simulink library "IOBlock_Library_TTC580"  (R2021a)
settings: Solver=ode45  StartTime=0.0  StopTime=10.0  RelTol=1e-3
PreLoadFcn:
  | addpath(genpath(fileparts(which('IOBlock_Library_TTC580'))));
  | %addpath(genpath(fileparts(which('IOBlock_Library_TTC580.mdl'))))
  | try
  | addpath(genpath([fileparts(which('IOBlock_Library_TTC580')),'\..\DBC_Importer']));
  | addpath(genpath([fileparts(which('IOBlock_Library_TTC580')),'\..\EEPROM_Importer']));
  | addpath(genpath([fileparts(which('IOBlock_Library_TTC580')),'\..\UserDoc']));
  | catch
  | warning('IOBlock_Library_TTC580: add path to DBC_Importer and EEPROM_Importer manually');
  | end
  | try
  | if exist('..\CustomPackage\scripts\OpenAllPackages.m','file')
  |      run('..\CustomPackage\scripts\OpenAllPackages.m'); %always available, ggf. empty
  | end
  | catch
  | warning('A problem occurred opening automatically the CustomPackage. Please open libraries manually');
  | end
  | try
  | set_param(0,'EditorSmartEditingHotParam','off');
  | catch
  | warning('Simlink preferences for ''Edit key parameter when adding new blocks'' needs to be unchecked manually');
  | end
undefined symbols (not defined in the file or in its folder): ADC_Absolute_10V, ADC_Absolute_32V, ADC_Absolute_5V, ADC_BoardTemp, ADC_ChannelInit, ADC_Current, ADC_Get, ADC_K15_, ADC_Ratiometric_10V, ADC_Ratiometric_5V, ADC_Resistive, ADC_SensorSupply, ADC_UBAT, bit_packing, bit_unpacking, CAN_ConfigMsg, compare2error, compare2FET_PROT_REENABLE, crc32_calc_intern, CRC32_EEPROM_Read, CRC32_EEPROM_Write, DIAG_EnterSafestate, DIAG_Status, DIAG_Status_internal, EEPROM_Mirror, EEPROM_Read, EEPROM_Read_OffsetIn, EEPROM_Read_Raw, EEPROM_Write, EEPROM_Write_OffsetIn, EEPROM_Write_Raw, EnterSafestate, FPU_Handler, Get_DI, Get_DI_VarThreshold, Get_K15_, Get_Pulse_Freq_Curr, Get_Pulse_Freq_Volt, Get_WakeUp, GetDateAndTime, IO_ADC_ResetProtection, IO_Blk_Lib_TTC500, IO_CAN_ReadMsg, IO_CAN_WriteMsg, IO_DI_Get, IO_DI_Init, IO_DI_Init_Var, IO_DO_GetCur, IO_DO_GetVoltage, IO_DO_Init, IO_DO_ResetProtection, IO_DO_Set, IO_Driver_GetSerialNumber, IO_Driver_GetVersionOfDriver, IO_Driver_GetVersionOfFPGA, IO_EEPROM_GetStatus, IO_EEPROM_Init, IO_EEPROM_Read_raw, IO_EEPROM_Write, IO_EEPROM_Write_OffsetIn ... (+73)
libraries: simulink x43
(part 8 of 18)

== system IOBlock_Library_TTC580/ADC Blocks TTC580 IOlib/ADC_UBAT ==
  ADC_ChannelInit : Subsystem  LoadFcn=|  mask(ADC_ChannelInit_Code){SampleTime=-1, ttlib=IO_Blk_Lib_TTC500, ttDescription=ADC_ChannelInit, tt_iolib_version=0.19, adc_channel=adc_channel, adc_type=adc_type, range=range, pupd=pupd, sensor_supply=sensor_supply, safety_conf=NULL}
      | try
      | %
      | %Upgrade Information - standard BEGIN
      | new_color = 'blue';
      | new_ver = '0.19';
      | act_ver = get_param(gcb,'tt_iolib_version');
      | if not(strcmp(act_ver,new_ver))
      |     disp(['Upgrade block: ',gcb,char(10),'       Version: ',act_ver,' -> ',new_ver]);
      |     %switch - case for specific upgrade information e.g. additional parameter required 
      |     %Change appearance and version information
      |     set_param(gcb,'ForegroundColor',new_color);
      |     set_param(gcb,'tt_iolib_version',new_ver);
      | end
      | %Upgrade Information - standard END
      | catch
      | %Standard catch section BEGIN 
      | disp(' ');
      | disp('------------------------------------------------------------');
      | disp('An error occurred in a callback of the TTC580-BlockLib.');
      | disp(['Please check the parameters in the mask of ',gcb]);
      | disp('If you do not encounter any violations, then please '); 
      | disp('copy the following lines and report this to support@ttcontrol.com ');
      | disp('<< begin of error message dump >>');
      | disp(['Version of TTC580-BlockLib: ', get_param(gcb,'tt_iolib_version')]);
      | disp(get_param(gcb,'ttDescription'));
      | disp(gcb);
      | x=lasterror;disp(x.message);
      | disp(get_param(gcb,'MaskValues'));
      | disp(version);
      | disp(computer);
      | disp('<< end of error message dump >>');
      | disp('------------------------------------------------------------');
      | disp(' ');
      | %Standard catch section END
      | end
      mask help: Setup one ADC channel.
      mask init:
      | %
      settings: CopyFcn=%deleted
      mask Help: web(which('IO_ADC.h'))
      mask Callback adc_channel: %
      mask Callback adc_type: %
      mask Callback range: %
      mask Callback pupd: %
      mask Callback sensor_supply: %
      mask Callback safety_conf: %
  ADC_Get : Subsystem  LoadFcn=|  mask(ADC_Get_Code){SampleTime=-1, ttlib=IO_Blk_Lib_TTC500, ttDescription=ADC_Get, tt_iolib_version=0.19, adc_channel=adc_channel}
      | try
      | %
      | %Upgrade Information - standard BEGIN
      | new_color = 'blue';
      | new_ver = '0.19';
      | act_ver = get_param(gcb,'tt_iolib_version');
      | if not(strcmp(act_ver,new_ver))
      |     disp(['Upgrade block: ',gcb,char(10),'       Version: ',act_ver,' -> ',new_ver]);
      |     %switch - case for specific upgrade information e.g. additional parameter required 
      |     %Change appearance and version information
      |     set_param(gcb,'ForegroundColor',new_color);
      |     set_param(gcb,'tt_iolib_version',new_ver);
      | end
      | %Upgrade Information - standard END
      | catch
      | %Standard catch section BEGIN 
      | disp(' ');
      | disp('------------------------------------------------------------');
      | disp('An error occurred in a callback of the TTC580-BlockLib.');
      | disp(['Please check the parameters in the mask of ',gcb]);
      | disp('If you do not encounter any violations, then please '); 
      | disp('copy the following lines and report this to support@ttcontrol.com ');
      | disp('<< begin of error message dump >>');
      | disp(['Version of TTC580-BlockLib: ', get_param(gcb,'tt_iolib_version')]);
      | disp(get_param(gcb,'ttDescription'));
      | disp(gcb);
      | x=lasterror;disp(x.message);
      | disp(get_param(gcb,'MaskValues'));
      | disp(version);
      | disp(computer);
      | disp('<< end of error message dump >>');
      | disp('------------------------------------------------------------');
      | disp(' ');
      | %Standard catch section END
      | end
      mask help: Returns the value of the given ADC channel.
      mask init:
      | %
      settings: CopyFcn=%deleted
      mask Help: web(which('IO_ADC.h'))
      mask Callback adc_channel: %
  PWM_Init : Terminator
  PWM_Init1 : Terminator
  ErrorCode : Outport  VectorParamsAs1DForOutWhenUnconnected=off
  adc_value : Outport  Port=2  VectorParamsAs1DForOutWhenUnconnected=off
  wires:
  ADC_ChannelInit/1(ErrorCode) -> PWM_Init/1
  ADC_Get/3(fresh) -> PWM_Init1/1
  ADC_Get/1(ErrorCode) -> ErrorCode/1
  ADC_Get/2(adc_value) -> adc_value/1

== system IOBlock_Library_TTC580/CAN  Blocks TTC580 IOlib/ReadMsg_CAN ==
  note: Used as link in CAN-dbc Import Template
  note: IO_ErrorTypes may be exported
      | by adding Outports manually
  CAN_ConfigMsg : Subsystem  LoadFcn=|  mask(CAN_ConfigMsg_Code){SampleTime=-1, ttlib=IO_Blk_Lib_TTC500, ttDescription=CAN_ConfigMsg, tt_iolib_version=0.19, channel=channel, mode=mode, id_format=(id_format-1) %PopupNr - 1, id=id, ac_mask=['0x',dec2hex((id_format==1)*hex2dec('7FF')+(id_format==2)*hex2dec('1FFFFFFF')),'U']; %id_format = PopupNr}
      | try
      | %
      | %Upgrade Information - standard BEGIN
      | new_color = 'blue';
      | new_ver = '0.19';
      | act_ver = get_param(gcb,'tt_iolib_version');
      | if not(strcmp(act_ver,new_ver))
      |     disp(['Upgrade block: ',gcb,char(10),'       Version: ',act_ver,' -> ',new_ver]);
      |     %switch - case for specific upgrade information e.g. additional parameter required 
      |     %Change appearance and version information
      |     set_param(gcb,'ForegroundColor',new_color);
      |     set_param(gcb,'tt_iolib_version',new_ver);
      | end
      | %Upgrade Information - standard END
      | catch
      | %Standard catch section BEGIN 
      | disp(' ');
      | disp('------------------------------------------------------------');
      | disp('An error occurred in a callback of the TTC580-BlockLib.');
      | disp(['Please check the parameters in the mask of ',gcb]);
      | disp('If you do not encounter any violations, then please '); 
      | disp('copy the following lines and report this to support@ttcontrol.com ');
      | disp('<< begin of error message dump >>');
      | disp(['Version of TTC580-BlockLib: ', get_param(gcb,'tt_iolib_version')]);
      | disp(get_param(gcb,'ttDescription'));
      | disp(gcb);
      | x=lasterror;disp(x.message);
      | disp(get_param(gcb,'MaskValues'));
      | disp(version);
      | disp(computer);
      | disp('<< end of error message dump >>');
      | disp('------------------------------------------------------------');
      | disp(' ');
      | %Standard catch section END
      | end
      mask help: Configures a message object for the given CAN channel.
      mask init:
      | %
      settings: CopyFcn=%deleted
      mask Help: web(which('IO_CAN.h'))
      mask Callback channel: %
      mask Callback mode: %
      mask Callback id_format: %
      mask Callback id: %
      mask Callback ac_mask: %
  IO_CAN_ReadMsg : Subsystem  LoadFcn=|  mask(IO_CAN_ReadMsg_Code){SampleTime=-1, ttlib=IO_Blk_Lib_TTC500, ttDescription=IO_CAN_ReadMsg, tt_iolib_version=0.19}
      | try
      | %
      | %Upgrade Information - standard BEGIN
      | new_color = 'blue';
      | new_ver = '0.19';
      | act_ver = get_param(gcb,'tt_iolib_version');
      | if not(strcmp(act_ver,new_ver))
      |     disp(['Upgrade block: ',gcb,char(10),'       Version: ',act_ver,' -> ',new_ver]);
      |     %switch - case for specific upgrade information e.g. additional parameter required 
      |     %Change appearance and version information
      |     set_param(gcb,'ForegroundColor',new_color);
      |     set_param(gcb,'tt_iolib_version',new_ver);
      | end
      | %Upgrade Information - standard END
      | catch
      | %Standard catch section BEGIN 
      | disp(' ');
      | disp('------------------------------------------------------------');
      | disp('An error occurred in a callback of the TTC580-BlockLib.');
      | disp(['Please check the parameters in the mask of ',gcb]);
      | disp('If you do not encounter any violations, then please '); 
      | disp('copy the following lines and report this to support@ttcontrol.com ');
      | disp('<< begin of error message dump >>');
      | disp(['Version of TTC580-BlockLib: ', get_param(gcb,'tt_iolib_version')]);
      | disp(get_param(gcb,'ttDescription'));
      | disp(gcb);
      | x=lasterror;disp(x.message);
      | disp(get_param(gcb,'MaskValues'));
      | disp(version);
      | disp(computer);
      | disp('<< end of error message dump >>');
      | disp('------------------------------------------------------------');
      | disp(' ');
      | %Standard catch section END
      | end
      mask help: Reads a message from a given message object.
      mask init:
      | %
      settings: CopyFcn=%deleted
      mask Help: web(which('IO_CAN.h'))
  Terminator{2,6..8} (4 alike) : Terminator
  Read_Error : Outport  VectorParamsAs1DForOutWhenUnconnected=off
  data : Outport  Port=2  VectorParamsAs1DForOutWhenUnconnected=off
  wires:
  CAN_ConfigMsg/2(handle) -> IO_CAN_ReadMsg/1(handle)
  IO_CAN_ReadMsg/2(buffer_data) -> data/1
  IO_CAN_ReadMsg/5(buffer_id) -> Terminator6/1
  IO_CAN_ReadMsg/4(buffer_id_format) -> Terminator7/1
  IO_CAN_ReadMsg/3(buffer_length) -> Terminator8/1
  CAN_ConfigMsg/1(ErrorCode) -> Terminator2/1
  IO_CAN_ReadMsg/1(ErrorCode) -> Read_Error/1

== system IOBlock_Library_TTC580/CAN  Blocks TTC580 IOlib/ReadMsg_CAN_derated ==
  note: IO_ErrorTypes may be exported
      | by adding Outports manually
  CAN_ConfigMsg : Subsystem  LoadFcn=|  mask(CAN_ConfigMsg_Code){SampleTime=-1, ttlib=IO_Blk_Lib_TTC500, ttDescription=CAN_ConfigMsg, tt_iolib_version=0.19, channel=channel, mode=mode, id_format=(id_format-1) %PopupNr - 1, id=id, ac_mask=['0x',dec2hex((id_format==1)*hex2dec('7FF')+(id_format==2)*hex2dec('1FFFFFFF')),'U']; %id_format = PopupNr}
      | try
      | %
      | %Upgrade Information - standard BEGIN
      | new_color = 'blue';
      | new_ver = '0.19';
      | act_ver = get_param(gcb,'tt_iolib_version');
      | if not(strcmp(act_ver,new_ver))
      |     disp(['Upgrade block: ',gcb,char(10),'       Version: ',act_ver,' -> ',new_ver]);
      |     %switch - case for specific upgrade information e.g. additional parameter required 
      |     %Change appearance and version information
      |     set_param(gcb,'ForegroundColor',new_color);
      |     set_param(gcb,'tt_iolib_version',new_ver);
      | end
      | %Upgrade Information - standard END
      | catch
      | %Standard catch section BEGIN 
      | disp(' ');
      | disp('------------------------------------------------------------');
      | disp('An error occurred in a callback of the TTC580-BlockLib.');
      | disp(['Please check the parameters in the mask of ',gcb]);
      | disp('If you do not encounter any violations, then please '); 
      | disp('copy the following lines and report this to support@ttcontrol.com ');
      | disp('<< begin of error message dump >>');
      | disp(['Version of TTC580-BlockLib: ', get_param(gcb,'tt_iolib_version')]);
      | disp(get_param(gcb,'ttDescription'));
      | disp(gcb);
      | x=lasterror;disp(x.message);
      | disp(get_param(gcb,'MaskValues'));
      | disp(version);
      | disp(computer);
      | disp('<< end of error message dump >>');
      | disp('------------------------------------------------------------');
      | disp(' ');
      | %Standard catch section END
      | end
      mask help: Configures a message object for the given CAN channel.
      mask init:
      | %
      settings: CopyFcn=%deleted
      mask Help: web(which('IO_CAN.h'))
      mask Callback channel: %
      mask Callback mode: %
      mask Callback id_format: %
      mask Callback id: %
      mask Callback ac_mask: %
  IO_CAN_ReadMsg_x : Subsystem  LoadFcn=|  mask(IO_CAN_ReadMsg_Code){SampleTime=-1, ttlib=IO_Blk_Lib_TTC500, ttDescription=IO_CAN_ReadMsg, tt_iolib_version=0.19}
      | try
      | %
      | %Upgrade Information - standard BEGIN
      | new_color = 'blue';
      | new_ver = '0.19';
      | act_ver = get_param(gcb,'tt_iolib_version');
      | if not(strcmp(act_ver,new_ver))
      |     disp(['Upgrade block: ',gcb,char(10),'       Version: ',act_ver,' -> ',new_ver]);
      |     %switch - case for specific upgrade information e.g. additional parameter required 
      |     %Change appearance and version information
      |     set_param(gcb,'ForegroundColor',new_color);
      |     set_param(gcb,'tt_iolib_version',new_ver);
      | end
      | %Upgrade Information - standard END
      | catch
      | %Standard catch section BEGIN 
      | disp(' ');
      | disp('------------------------------------------------------------');
      | disp('An error occurred in a callback of the TTC580-BlockLib.');
      | disp(['Please check the parameters in the mask of ',gcb]);
      | disp('If you do not encounter any violations, then please '); 
      | disp('copy the following lines and report this to support@ttcontrol.com ');
      | disp('<< begin of error message dump >>');
      | disp(['Version of TTC580-BlockLib: ', get_param(gcb,'tt_iolib_version')]);
      | disp(get_param(gcb,'ttDescription'));
      | disp(gcb);
      | x=lasterror;disp(x.message);
      | disp(get_param(gcb,'MaskValues'));
      | disp(version);
      | disp(computer);
      | disp('<< end of error message dump >>');
      | disp('------------------------------------------------------------');
      | disp(' ');
      | %Standard catch section END
      | end
      mask help: Reads a message from a given message object.
      mask init:
      | %
      settings: CopyFcn=%deleted
      mask Help: web(which('IO_CAN.h'))
  Terminator{2,6..8} (4 alike) : Terminator
  Trigger : Subsystem  mask(Derate Trigger){derate=derate}
      mask help: derate "n": every n-th cylce a trigger is submitted
  Read_Error_debcd : Outport  VectorParamsAs1DForOutWhenUnconnected=off
  data : Outport  Port=2  VectorParamsAs1DForOutWhenUnconnected=off
  wires:
  IO_CAN_ReadMsg_x/1(ErrorCode) -> Read_Error_debcd/1
  CAN_ConfigMsg/1(ErrorCode) -> Terminator2/1
  IO_CAN_ReadMsg_x/3(buffer_length) -> Terminator8/1
  IO_CAN_ReadMsg_x/4(buffer_id_format) -> Terminator7/1
  IO_CAN_ReadMsg_x/5(buffer_id) -> Terminator6/1
  IO_CAN_ReadMsg_x/2(buffer_data) -> data/1
  CAN_ConfigMsg/2(handle) -> IO_CAN_ReadMsg_x/1(handle)
  Trigger/1(Trigger) -> IO_CAN_ReadMsg_x/Enable

== system IOBlock_Library_TTC580/CAN  Blocks TTC580 IOlib/WriteMsg_CAN ==
  note: IO_ErrorTypes may be exported
      | by adding Outports manually
  note: Used as link in CAN-dbc Import Template
  data : Inport
  CAN_ConfigMsg : Subsystem  LoadFcn=|  mask(CAN_ConfigMsg_Code){SampleTime=-1, ttlib=IO_Blk_Lib_TTC500, ttDescription=CAN_ConfigMsg, tt_iolib_version=0.19, channel=channel, mode=mode, id_format=(id_format-1) %PopupNr - 1, id=id, ac_mask=['0x',dec2hex((id_format==1)*hex2dec('7FF')+(id_format==2)*hex2dec('1FFFFFFF')),'U']; %id_format = PopupNr}
      | try
      | %
      | %Upgrade Information - standard BEGIN
      | new_color = 'blue';
      | new_ver = '0.19';
      | act_ver = get_param(gcb,'tt_iolib_version');
      | if not(strcmp(act_ver,new_ver))
      |     disp(['Upgrade block: ',gcb,char(10),'       Version: ',act_ver,' -> ',new_ver]);
      |     %switch - case for specific upgrade information e.g. additional parameter required 
      |     %Change appearance and version information
      |     set_param(gcb,'ForegroundColor',new_color);
      |     set_param(gcb,'tt_iolib_version',new_ver);
      | end
      | %Upgrade Information - standard END
      | catch
      | %Standard catch section BEGIN 
      | disp(' ');
      | disp('------------------------------------------------------------');
      | disp('An error occurred in a callback of the TTC580-BlockLib.');
      | disp(['Please check the parameters in the mask of ',gcb]);
      | disp('If you do not encounter any violations, then please '); 
      | disp('copy the following lines and report this to support@ttcontrol.com ');
      | disp('<< begin of error message dump >>');
      | disp(['Version of TTC580-BlockLib: ', get_param(gcb,'tt_iolib_version')]);
      | disp(get_param(gcb,'ttDescription'));
      | disp(gcb);
      | x=lasterror;disp(x.message);
      | disp(get_param(gcb,'MaskValues'));
      | disp(version);
      | disp(computer);
      | disp('<< end of error message dump >>');
      | disp('------------------------------------------------------------');
      | disp(' ');
      | %Standard catch section END
      | end
      mask help: Configures a message object for the given CAN channel.
      mask init:
      | %
      settings: CopyFcn=%deleted
      mask Help: web(which('IO_CAN.h'))
      mask Callback channel: %
      mask Callback mode: %
      mask Callback id_format: %
      mask Callback id: %
      mask Callback ac_mask: %
  IO_CAN_WriteMsg : Subsystem  LoadFcn=|  mask(IO_CAN_WriteMsg_Code){SampleTime=-1, ttlib=IO_Blk_Lib_TTC500, ttDescription=IO_CAN_WriteMsg, tt_iolib_version=0.19}
      | try
      | %
      | %Upgrade Information - standard BEGIN
      | new_color = 'blue';
      | new_ver = '0.19';
      | act_ver = get_param(gcb,'tt_iolib_version');
      | if not(strcmp(act_ver,new_ver))
      |     disp(['Upgrade block: ',gcb,char(10),'       Version: ',act_ver,' -> ',new_ver]);
      |     %switch - case for specific upgrade information e.g. additional parameter required 
      |     %Change appearance and version information
      |     set_param(gcb,'ForegroundColor',new_color);
      |     set_param(gcb,'tt_iolib_version',new_ver);
      | end
      | %Upgrade Information - standard END
      | catch
      | %Standard catch section BEGIN 
      | disp(' ');
      | disp('------------------------------------------------------------');
      | disp('An error occurred in a callback of the TTC580-BlockLib.');
      | disp(['Please check the parameters in the mask of ',gcb]);
      | disp('If you do not encounter any violations, then please '); 
      | disp('copy the following lines and report this to support@ttcontrol.com ');
      | disp('<< begin of error message dump >>');
      | disp(['Version of TTC580-BlockLib: ', get_param(gcb,'tt_iolib_version')]);
      | disp(get_param(gcb,'ttDescription'));
      | disp(gcb);
      | x=lasterror;disp(x.message);
      | disp(get_param(gcb,'MaskValues'));
      | disp(version);
      | disp(computer);
      | disp('<< end of error message dump >>');
      | disp('------------------------------------------------------------');
      | disp(' ');
      | %Standard catch section END
      | end
      mask help: Transmits a CAN message, using the given channel and message object.
      mask init:
      | %
      settings: CopyFcn=%deleted
      mask Help: web(which('IO_CAN.h'))
  Terminator2 : Terminator
  id_TX : Constant  Value=id  OutDataTypeStr=uint32
  id_format_TX : Constant  Value=(id_format - 1) %=PopupEntryNr - 1  OutDataTypeStr=Inherit: Inherit via back propagation
  length_TX : Constant  Value=length  OutDataTypeStr=Inherit: Inherit via back propagation
  Write_Error : Outport  VectorParamsAs1DForOutWhenUnconnected=off
  wires:
  CAN_ConfigMsg/1(ErrorCode) -> Terminator2/1
  IO_CAN_WriteMsg/1(ErrorCode) -> Write_Error/1
  CAN_ConfigMsg/2(handle) -> IO_CAN_WriteMsg/1(handle)
  data/1 -> IO_CAN_WriteMsg/2(buffer_data)
  length_TX/1 -> IO_CAN_WriteMsg/3(buffer_length)
  id_format_TX/1 -> IO_CAN_WriteMsg/4(buffer_id_format)
  id_TX/1 -> IO_CAN_WriteMsg/5(buffer_id)

== system IOBlock_Library_TTC580/CAN  Blocks TTC580 IOlib/WriteMsg_CAN_derated ==
  note: IO_ErrorTypes may be exported
      | by adding Outports manually
  data : Inport
  CAN_ConfigMsg : Subsystem  LoadFcn=|  mask(CAN_ConfigMsg_Code){SampleTime=-1, ttlib=IO_Blk_Lib_TTC500, ttDescription=CAN_ConfigMsg, tt_iolib_version=0.19, channel=channel, mode=mode, id_format=(id_format-1) %PopupNr - 1, id=id, ac_mask=['0x',dec2hex((id_format==1)*hex2dec('7FF')+(id_format==2)*hex2dec('1FFFFFFF')),'U']; %id_format = PopupNr}
      | try
      | %
      | %Upgrade Information - standard BEGIN
      | new_color = 'blue';
      | new_ver = '0.19';
      | act_ver = get_param(gcb,'tt_iolib_version');
      | if not(strcmp(act_ver,new_ver))
      |     disp(['Upgrade block: ',gcb,char(10),'       Version: ',act_ver,' -> ',new_ver]);
      |     %switch - case for specific upgrade information e.g. additional parameter required 
      |     %Change appearance and version information
      |     set_param(gcb,'ForegroundColor',new_color);
      |     set_param(gcb,'tt_iolib_version',new_ver);
      | end
      | %Upgrade Information - standard END
      | catch
      | %Standard catch section BEGIN 
      | disp(' ');
      | disp('------------------------------------------------------------');
      | disp('An error occurred in a callback of the TTC580-BlockLib.');
      | disp(['Please check the parameters in the mask of ',gcb]);
      | disp('If you do not encounter any violations, then please '); 
      | disp('copy the following lines and report this to support@ttcontrol.com ');
      | disp('<< begin of error message dump >>');
      | disp(['Version of TTC580-BlockLib: ', get_param(gcb,'tt_iolib_version')]);
      | disp(get_param(gcb,'ttDescription'));
      | disp(gcb);
      | x=lasterror;disp(x.message);
      | disp(get_param(gcb,'MaskValues'));
      | disp(version);
      | disp(computer);
      | disp('<< end of error message dump >>');
      | disp('------------------------------------------------------------');
      | disp(' ');
      | %Standard catch section END
      | end
      mask help: Configures a message object for the given CAN channel.
      mask init:
      | %
      settings: CopyFcn=%deleted
      mask Help: web(which('IO_CAN.h'))
      mask Callback channel: %
      mask Callback mode: %
      mask Callback id_format: %
      mask Callback id: %
      mask Callback ac_mask: %
  IO_CAN_WriteMsg_x : Subsystem  LoadFcn=|  mask(IO_CAN_WriteMsg_Code){SampleTime=-1, ttlib=IO_Blk_Lib_TTC500, ttDescription=IO_CAN_WriteMsg, tt_iolib_version=0.19}
      | try
      | %
      | %Upgrade Information - standard BEGIN
      | new_color = 'blue';
      | new_ver = '0.19';
      | act_ver = get_param(gcb,'tt_iolib_version');
      | if not(strcmp(act_ver,new_ver))
      |     disp(['Upgrade block: ',gcb,char(10),'       Version: ',act_ver,' -> ',new_ver]);
      |     %switch - case for specific upgrade information e.g. additional parameter required 
      |     %Change appearance and version information
      |     set_param(gcb,'ForegroundColor',new_color);
      |     set_param(gcb,'tt_iolib_version',new_ver);
      | end
      | %Upgrade Information - standard END
      | catch
      | %Standard catch section BEGIN 
      | disp(' ');
      | disp('------------------------------------------------------------');
      | disp('An error occurred in a callback of the TTC580-BlockLib.');
      | disp(['Please check the parameters in the mask of ',gcb]);
      | disp('If you do not encounter any violations, then please '); 
      | disp('copy the following lines and report this to support@ttcontrol.com ');
      | disp('<< begin of error message dump >>');
      | disp(['Version of TTC580-BlockLib: ', get_param(gcb,'tt_iolib_version')]);
      | disp(get_param(gcb,'ttDescription'));
      | disp(gcb);
      | x=lasterror;disp(x.message);
      | disp(get_param(gcb,'MaskValues'));
      | disp(version);
      | disp(computer);
      | disp('<< end of error message dump >>');
      | disp('------------------------------------------------------------');
      | disp(' ');
      | %Standard catch section END
      | end
      mask help: Transmits a CAN message, using the given channel and message object.
      mask init:
      | %
      settings: CopyFcn=%deleted
      mask Help: web(which('IO_CAN.h'))
  Terminator2 : Terminator
  Trigger : Subsystem  mask(Derate Trigger){derate=derate}
      mask help: derate "n": every n-th cylce a trigger is submitted
  id_TX : Constant  Value=id  OutDataTypeStr=uint32
  id_format_TX : Constant  Value=(id_format - 1) %=PopupEntryNr - 1  OutDataTypeStr=Inherit: Inherit via back propagation
  length_TX : Constant  Value=length  OutDataTypeStr=Inherit: Inherit via back propagation
  Write_Error : Outport  VectorParamsAs1DForOutWhenUnconnected=off
  wires:
  Trigger/1(Trigger) -> IO_CAN_WriteMsg_x/Enable
  id_TX/1 -> IO_CAN_WriteMsg_x/5(buffer_id)
  id_format_TX/1 -> IO_CAN_WriteMsg_x/4(buffer_id_format)
  length_TX/1 -> IO_CAN_WriteMsg_x/3(buffer_length)
  data/1 -> IO_CAN_WriteMsg_x/2(buffer_data)
  CAN_ConfigMsg/2(handle) -> IO_CAN_WriteMsg_x/1(handle)
  IO_CAN_WriteMsg_x/1(ErrorCode) -> Write_Error/1
  CAN_ConfigMsg/1(ErrorCode) -> Terminator2/1

== system IOBlock_Library_TTC580/CAN  Blocks TTC580 IOlib/bit_packing ==
  Data_in : Inport
  bit_packing_s : S-Function  FunctionName=bit_packing_s  Parameters=SampleTime,Endianness,Format,Inversion,Startbit,Width_bits,Factor,Offset  SFunctionDeploymentMode=off  EnableBusSupport=off
  Data_out : Outport  VectorParamsAs1DForOutWhenUnconnected=off
  wires:
  bit_packing_s/1 -> Data_out/1
  Data_in/1 -> bit_packing_s/1

== system IOBlock_Library_TTC580/CAN  Blocks TTC580 IOlib/bit_unpacking ==
  Data_in : Inport
  bit_unpacking_s : S-Function  FunctionName=bit_unpacking_s  Parameters=SampleTime,Endianness,Format,Inversion,Startbit,Width_bits,Factor,Offset  SFunctionDeploymentMode=off  EnableBusSupport=off
  Data_out : Outport  VectorParamsAs1DForOutWhenUnconnected=off
  wires:
  bit_unpacking_s/1 -> Data_out/1
  Data_in/1 -> bit_unpacking_s/1

== system IOBlock_Library_TTC580/DIO Blocks TTC580 IOlib/Get_DI ==
  IO_DI_Get : Subsystem  LoadFcn=|  mask(IO_DI_Get_Code){SampleTime=-1, ttlib=IO_Blk_Lib_TTC500, ttDescription=IO_DI_Get, tt_iolib_version=0.19, di_channel=di_channel}
      | try
      | %
      | %Upgrade Information - standard BEGIN
      | new_color = 'blue';
      | new_ver = '0.19';
      | act_ver = get_param(gcb,'tt_iolib_version');
      | if not(strcmp(act_ver,new_ver))
      |     disp(['Upgrade block: ',gcb,char(10),'       Version: ',act_ver,' -> ',new_ver]);
      |     %switch - case for specific upgrade information e.g. additional parameter required 
      |     %Change appearance and version information
      |     set_param(gcb,'ForegroundColor',new_color);
      |     set_param(gcb,'tt_iolib_version',new_ver);
      | end
      | %Upgrade Information - standard END
      | catch
      | %Standard catch section BEGIN 
      | disp(' ');
      | disp('------------------------------------------------------------');
      | disp('An error occurred in a callback of the TTC580-BlockLib.');
      | disp(['Please check the parameters in the mask of ',gcb]);
      | disp('If you do not encounter any violations, then please '); 
      | disp('copy the following lines and report this to support@ttcontrol.com ');
      | disp('<< begin of error message dump >>');
      | disp(['Version of TTC580-BlockLib: ', get_param(gcb,'tt_iolib_version')]);
      | disp(get_param(gcb,'ttDescription'));
      | disp(gcb);
      | x=lasterror;disp(x.message);
      | disp(get_param(gcb,'MaskValues'));
      | disp(version);
      | disp(computer);
      | disp('<< end of error message dump >>');
      | disp('------------------------------------------------------------');
      | disp(' ');
      | %Standard catch section END
      | end
      mask help: Gets the value of a digital input.
      mask init:
      | %
      settings: CopyFcn=%deleted
      mask Help: web(which('IO_DIO.h'))
      mask Callback di_channel: %
  IO_DI_Init : Subsystem  LoadFcn=|  mask(IO_DI_Init_Code){SampleTime=-1, ttlib=IO_Blk_Lib_TTC500, ttDescription=IO_DI_Init, tt_iolib_version=0.19, di_channel=di_channel, pupd=pupd, limits=NULL}
      | try
      | %
      | %Upgrade Information - standard BEGIN
      | new_color = 'blue';
      | new_ver = '0.19';
      | act_ver = get_param(gcb,'tt_iolib_version');
      | if not(strcmp(act_ver,new_ver))
      |     disp(['Upgrade block: ',gcb,char(10),'       Version: ',act_ver,' -> ',new_ver]);
      |     %switch - case for specific upgrade information e.g. additional parameter required 
      |     %Change appearance and version information
      |     set_param(gcb,'ForegroundColor',new_color);
      |     set_param(gcb,'tt_iolib_version',new_ver);
      | end
      | %Upgrade Information - standard END
      | catch
      | %Standard catch section BEGIN 
      | disp(' ');
      | disp('------------------------------------------------------------');
      | disp('An error occurred in a callback of the TTC580-BlockLib.');
      | disp(['Please check the parameters in the mask of ',gcb]);
      | disp('If you do not encounter any violations, then please '); 
      | disp('copy the following lines and report this to support@ttcontrol.com ');
      | disp('<< begin of error message dump >>');
      | disp(['Version of TTC580-BlockLib: ', get_param(gcb,'tt_iolib_version')]);
      | disp(get_param(gcb,'ttDescription'));
      | disp(gcb);
      | x=lasterror;disp(x.message);
      | disp(get_param(gcb,'MaskValues'));
      | disp(version);
      | disp(computer);
      | disp('<< end of error message dump >>');
      | disp('------------------------------------------------------------');
      | disp(' ');
      | %Standard catch section END
      | end
      mask help: Setup a digital input.
      mask init:
      | %
      settings: CopyFcn=%deleted
      mask Help: web(which('IO_DIO.h'))
      mask Callback di_channel: %
      mask Callback pupd: %
      mask Callback limits: %
  Terminator : Terminator
  ErrorCode : Outport  VectorParamsAs1DForOutWhenUnconnected=off
  di_value : Outport  Port=2  VectorParamsAs1DForOutWhenUnconnected=off
  wires:
  IO_DI_Get/2(di_value) -> di_value/1
  IO_DI_Get/1(ErrorCode) -> ErrorCode/1
  IO_DI_Init/1(ErrorCode) -> Terminator/1

== system IOBlock_Library_TTC580/DIO Blocks TTC580 IOlib/Get_DI_VarThreshold ==
  IO_DI_Get : Subsystem  LoadFcn=|  mask(IO_DI_Get_Code){SampleTime=-1, ttlib=IO_Blk_Lib_TTC500, ttDescription=IO_DI_Get, tt_iolib_version=0.19, di_channel=di_channel}
      | try
      | %
      | %Upgrade Information - standard BEGIN
      | new_color = 'blue';
      | new_ver = '0.19';
      | act_ver = get_param(gcb,'tt_iolib_version');
      | if not(strcmp(act_ver,new_ver))
      |     disp(['Upgrade block: ',gcb,char(10),'       Version: ',act_ver,' -> ',new_ver]);
      |     %switch - case for specific upgrade information e.g. additional parameter required 
      |     %Change appearance and version information
      |     set_param(gcb,'ForegroundColor',new_color);
      |     set_param(gcb,'tt_iolib_version',new_ver);
      | end
      | %Upgrade Information - standard END
      | catch
      | %Standard catch section BEGIN 
      | disp(' ');
      | disp('------------------------------------------------------------');
      | disp('An error occurred in a callback of the TTC580-BlockLib.');
      | disp(['Please check the parameters in the mask of ',gcb]);
      | disp('If you do not encounter any violations, then please '); 
      | disp('copy the following lines and report this to support@ttcontrol.com ');
      | disp('<< begin of error message dump >>');
      | disp(['Version of TTC580-BlockLib: ', get_param(gcb,'tt_iolib_version')]);
      | disp(get_param(gcb,'ttDescription'));
      | disp(gcb);
      | x=lasterror;disp(x.message);
      | disp(get_param(gcb,'MaskValues'));
      | disp(version);
      | disp(computer);
      | disp('<< end of error message dump >>');
      | disp('------------------------------------------------------------');
      | disp(' ');
      | %Standard catch section END
      | end
      mask help: Gets the value of a digital input.
      mask init:
      | %
      settings: CopyFcn=%deleted
      mask Help: web(which('IO_DIO.h'))
      mask Callback di_channel: %
  IO_DI_Init_Var : Subsystem  LoadFcn=|  mask(IO_DI_Init_Var_Code){SampleTime=-1, ttlib=IO_Blk_Lib_TTC500, ttDescription=IO_DI_Init_Var, tt_iolib_version=0.19, di_channel=di_channel, pupd=pupd, limits_low_thresh1=low_thresh1_mV, limits_low_thresh2=low_thresh2_mV, limits_high_thresh1=high_thresh1_mV, limits_high_thresh2=high_thresh2_mV}
      | try
      | %
      | %Upgrade Information - standard BEGIN
      | new_color = 'blue';
      | new_ver = '0.19';
      | act_ver = get_param(gcb,'tt_iolib_version');
      | if not(strcmp(act_ver,new_ver))
      |     disp(['Upgrade block: ',gcb,char(10),'       Version: ',act_ver,' -> ',new_ver]);
      |     %switch - case for specific upgrade information e.g. additional parameter required 
      |     %Change appearance and version information
      |     set_param(gcb,'ForegroundColor',new_color);
      |     set_param(gcb,'tt_iolib_version',new_ver);
      | end
      | %Upgrade Information - standard END
      | catch
      | %Standard catch section BEGIN 
      | disp(' ');
      | disp('------------------------------------------------------------');
      | disp('An error occurred in a callback of the TTC580-BlockLib.');
      | disp(['Please check the parameters in the mask of ',gcb]);
      | disp('If you do not encounter any violations, then please '); 
      | disp('copy the following lines and report this to support@ttcontrol.com ');
      | disp('<< begin of error message dump >>');
      | disp(['Version of TTC580-BlockLib: ', get_param(gcb,'tt_iolib_version')]);
      | disp(get_param(gcb,'ttDescription'));
      | disp(gcb);
      | x=lasterror;disp(x.message);
      | disp(get_param(gcb,'MaskValues'));
      | disp(version);
      | disp(computer);
      | disp('<< end of error message dump >>');
      | disp('------------------------------------------------------------');
      | disp(' ');
      | %Standard catch section END
      | end
      mask help: Setup a digital input with safety configuration.
      mask init:
      | %
      settings: CopyFcn=%deleted
      mask Help: web(which('IO_DIO.h'))
      mask Callback di_channel: %
      mask Callback pupd: %
      mask Callback limits_low_thresh1: %
      mask Callback limits_low_thresh2: %
      mask Callback limits_high_thresh1: %
      mask Callback limits_high_thresh2: %
  Terminator : Terminator
  ErrorCode : Outport  VectorParamsAs1DForOutWhenUnconnected=off
  di_value : Outport  Port=2  VectorParamsAs1DForOutWhenUnconnected=off
  wires:
  IO_DI_Get/2(di_value) -> di_value/1
  IO_DI_Get/1(ErrorCode) -> ErrorCode/1
  IO_DI_Init_Var/1(ErrorCode) -> Terminator/1

== system IOBlock_Library_TTC580/DIO Blocks TTC580 IOlib/Get_K15_ ==
  POWER_Get : Subsystem  LoadFcn=|  mask(POWER_Get_Code){SampleTime=-1, ttlib=IO_Blk_Lib_TTC500, ttDescription=POWER_Get, tt_iolib_version=0.19, pin=pin}
      | try
      | %
      | %Upgrade Information - standard BEGIN
      | new_color = 'blue';
      | new_ver = '0.19';
      | act_ver = get_param(gcb,'tt_iolib_version');
      | if not(strcmp(act_ver,new_ver))
      |     disp(['Upgrade block: ',gcb,char(10),'       Version: ',act_ver,' -> ',new_ver]);
      |     %switch - case for specific upgrade information e.g. additional parameter required 
      |     %Change appearance and version information
      |     set_param(gcb,'ForegroundColor',new_color);
      |     set_param(gcb,'tt_iolib_version',new_ver);
      | end
      | %Upgrade Information - standard END
      | catch
      | %Standard catch section BEGIN 
      | disp(' ');
      | disp('------------------------------------------------------------');
      | disp('An error occurred in a callback of the TTC580-BlockLib.');
      | disp(['Please check the parameters in the mask of ',gcb]);
      | disp('If you do not encounter any violations, then please '); 
      | disp('copy the following lines and report this to support@ttcontrol.com ');
      | disp('<< begin of error message dump >>');
      | disp(['Version of TTC580-BlockLib: ', get_param(gcb,'tt_iolib_version')]);
      | disp(get_param(gcb,'ttDescription'));
      | disp(gcb);
      | x=lasterror;disp(x.message);
      | disp(get_param(gcb,'MaskValues'));
      | disp(version);
      | disp(computer);
      | disp('<< end of error message dump >>');
      | disp('------------------------------------------------------------');
      | disp(' ');
      | %Standard catch section END
      | end
      mask help: Returns the current state of a POWER feature.
      mask init:
      | %
      settings: CopyFcn=%deleted
      mask Help: web(which('IO_POWER.h'))
      mask Callback pin: %
  ErrorCode : Outport  VectorParamsAs1DForOutWhenUnconnected=off
  state : Outport  Port=2  VectorParamsAs1DForOutWhenUnconnected=off
  wires:
  POWER_Get/2(state) -> state/1
  POWER_Get/1(ErrorCode) -> ErrorCode/1

== system IOBlock_Library_TTC580/DIO Blocks TTC580 IOlib/Get_WakeUp ==
  POWER_Get : Subsystem  LoadFcn=|  mask(POWER_Get_Code){SampleTime=-1, ttlib=IO_Blk_Lib_TTC500, ttDescription=POWER_Get, tt_iolib_version=0.19, pin=pin}
      | try
      | %
      | %Upgrade Information - standard BEGIN
      | new_color = 'blue';
      | new_ver = '0.19';
      | act_ver = get_param(gcb,'tt_iolib_version');
      | if not(strcmp(act_ver,new_ver))
      |     disp(['Upgrade block: ',gcb,char(10),'       Version: ',act_ver,' -> ',new_ver]);
      |     %switch - case for specific upgrade information e.g. additional parameter required 
      |     %Change appearance and version information
      |     set_param(gcb,'ForegroundColor',new_color);
      |     set_param(gcb,'tt_iolib_version',new_ver);
      | end
      | %Upgrade Information - standard END
      | catch
      | %Standard catch section BEGIN 
      | disp(' ');
      | disp('------------------------------------------------------------');
      | disp('An error occurred in a callback of the TTC580-BlockLib.');
      | disp(['Please check the parameters in the mask of ',gcb]);
      | disp('If you do not encounter any violations, then please '); 
      | disp('copy the following lines and report this to support@ttcontrol.com ');
      | disp('<< begin of error message dump >>');
      | disp(['Version of TTC580-BlockLib: ', get_param(gcb,'tt_iolib_version')]);
      | disp(get_param(gcb,'ttDescription'));
      | disp(gcb);
      | x=lasterror;disp(x.message);
      | disp(get_param(gcb,'MaskValues'));
      | disp(version);
      | disp(computer);
      | disp('<< end of error message dump >>');
      | disp('------------------------------------------------------------');
      | disp(' ');
      | %Standard catch section END
      | end
      mask help: Returns the current state of a POWER feature.
      mask init:
      | %
      settings: CopyFcn=%deleted
      mask Help: web(which('IO_POWER.h'))
      mask Callback pin: %
  ErrorCode : Outport  VectorParamsAs1DForOutWhenUnconnected=off
  state : Outport  Port=2  VectorParamsAs1DForOutWhenUnconnected=off
  wires:
  POWER_Get/2(state) -> state/1
  POWER_Get/1(ErrorCode) -> ErrorCode/1
